simulink model "model_compatible"  (Simulink 7.5)
(part 2 of 2)

  G_23802422_Kernkraftwerk_Isar/RConn2 -- _CN_77697810_380000_CN23802422/RConn2
  G_23802422_Kernkraftwerk_Isar/RConn3 -- _CN_77697810_380000_CN23802422/RConn3
  T_24976300_380000;220000;110000_Umspannwerk_Pleinting/LConn1 -- _CN_77697810_380000_CN_24976300_380000/RConn1
  T_24976300_380000;220000;110000_Umspannwerk_Pleinting/LConn2 -- _CN_77697810_380000_CN_24976300_380000/RConn2
  T_24976300_380000;220000;110000_Umspannwerk_Pleinting/LConn3 -- _CN_77697810_380000_CN_24976300_380000/RConn3
  Nfi_Oh_CN_24158385_220000_CN_26245195_220000/LConn1 -- T_24158385_220000;110000_Umspannwerk_Neufinsing/LConn1 -- Oberbachern___Neufinsing_CN_24158385_220000_CN_18629425_220000/LConn1 -- _CN_24158385_220000_CN_75865676_220000/LConn1 -- Neufinsing___Zolling_CN_24158385_220000_CN29122363/LConn1 -- Neufinsing___Zolling_CN_24158385_220000_CN_133342285_220000/RConn1
  Nfi_Oh_CN_24158385_220000_CN_26245195_220000/LConn2 -- T_24158385_220000;110000_Umspannwerk_Neufinsing/LConn2 -- Oberbachern___Neufinsing_CN_24158385_220000_CN_18629425_220000/LConn2 -- _CN_24158385_220000_CN_75865676_220000/LConn2 -- Neufinsing___Zolling_CN_24158385_220000_CN29122363/LConn2 -- Neufinsing___Zolling_CN_24158385_220000_CN_133342285_220000/RConn2
  Nfi_Oh_CN_24158385_220000_CN_26245195_220000/LConn3 -- T_24158385_220000;110000_Umspannwerk_Neufinsing/LConn3 -- Oberbachern___Neufinsing_CN_24158385_220000_CN_18629425_220000/LConn3 -- _CN_24158385_220000_CN_75865676_220000/LConn3 -- Neufinsing___Zolling_CN_24158385_220000_CN29122363/LConn3 -- Neufinsing___Zolling_CN_24158385_220000_CN_133342285_220000/RConn3
  Nfi_Oh_CN_24158385_220000_CN_26245195_220000/RConn1 -- T_26245195_380000;220000_Umspannwerk_Ottenhofen/RConn1 -- L_26245195/LConn1
  Nfi_Oh_CN_24158385_220000_CN_26245195_220000/RConn2 -- T_26245195_380000;220000_Umspannwerk_Ottenhofen/RConn2 -- L_26245195/LConn2
  Nfi_Oh_CN_24158385_220000_CN_26245195_220000/RConn3 -- T_26245195_380000;220000_Umspannwerk_Ottenhofen/RConn3 -- L_26245195/LConn3
  Oberbachern___Neufinsing_CN_24158385_220000_CN_18629425_220000/RConn1 -- T_18629425_380000;220000;110000_Umspannwerk_Oberbachern/RConn1 -- Oberbrunn___Oberbachern_CN_18629425_220000_CN_24237879_220000/LConn1
  Oberbachern___Neufinsing_CN_24158385_220000_CN_18629425_220000/RConn2 -- T_18629425_380000;220000;110000_Umspannwerk_Oberbachern/RConn2 -- Oberbrunn___Oberbachern_CN_18629425_220000_CN_24237879_220000/LConn2
  Oberbachern___Neufinsing_CN_24158385_220000_CN_18629425_220000/RConn3 -- T_18629425_380000;220000;110000_Umspannwerk_Oberbachern/RConn3 -- Oberbrunn___Oberbachern_CN_18629425_220000_CN_24237879_220000/LConn3
  T_75865676_220000_Umspannwerk_Marienberg/LConn1 -- _CN_24158385_220000_CN_75865676_220000/RConn1
  T_75865676_220000_Umspannwerk_Marienberg/LConn2 -- _CN_24158385_220000_CN_75865676_220000/RConn2
  T_75865676_220000_Umspannwerk_Marienberg/LConn3 -- _CN_24158385_220000_CN_75865676_220000/RConn3
  Neufinsing___Zolling_CN_24158385_220000_CN29122363/RConn1 -- G_29122363_Kraftwerk_Irsching/RConn1 -- _CN_18629425_380000_CN29122363/LConn1 -- Irsching___Raitersaich_CN_24768051_380000_CN29122363/LConn1 -- _CN_137602559_220000_CN29122363/LConn1
  Neufinsing___Zolling_CN_24158385_220000_CN29122363/RConn2 -- G_29122363_Kraftwerk_Irsching/RConn2 -- _CN_18629425_380000_CN29122363/LConn2 -- Irsching___Raitersaich_CN_24768051_380000_CN29122363/LConn2 -- _CN_137602559_220000_CN29122363/LConn2
  Neufinsing___Zolling_CN_24158385_220000_CN29122363/RConn3 -- G_29122363_Kraftwerk_Irsching/RConn3 -- _CN_18629425_380000_CN29122363/LConn3 -- Irsching___Raitersaich_CN_24768051_380000_CN29122363/LConn3 -- _CN_137602559_220000_CN29122363/LConn3
  T_78441561_380000;110000_Umspannwerk_Plattling/LConn1 -- Pleinting___Plattling___Schwandorf_CN_78441561_380000_CN_28956649_380000/LConn1
  T_78441561_380000;110000_Umspannwerk_Plattling/LConn2 -- Pleinting___Plattling___Schwandorf_CN_78441561_380000_CN_28956649_380000/LConn2
  T_78441561_380000;110000_Umspannwerk_Plattling/LConn3 -- Pleinting___Plattling___Schwandorf_CN_78441561_380000_CN_28956649_380000/LConn3
  Pleinting___Plattling___Schwandorf_CN_78441561_380000_CN_28956649_380000/RConn1 -- T_28956649_380000;220000;110000_Schwandorf/LConn1 -- Schwandorf___Etzenricht_CN_29084374_380000_CN_28956649_380000/LConn1
  Pleinting___Plattling___Schwandorf_CN_78441561_380000_CN_28956649_380000/RConn2 -- T_28956649_380000;220000;110000_Schwandorf/LConn2 -- Schwandorf___Etzenricht_CN_29084374_380000_CN_28956649_380000/LConn2
  Pleinting___Plattling___Schwandorf_CN_78441561_380000_CN_28956649_380000/RConn3 -- T_28956649_380000;220000;110000_Schwandorf/LConn3 -- Schwandorf___Etzenricht_CN_29084374_380000_CN_28956649_380000/LConn3
  LU_SIT_CN_24759324_220000_CN_133349218_220000/RConn1 -- T_24759324_220000;110000_Umspannwerk_Sittling/LConn1 -- Altheim___Sittling_CN_24759324_220000_CN_77694901_220000/RConn1 -- IN_SIT_CN_24759324_220000_CN_24768051_220000/LConn1
  LU_SIT_CN_24759324_220000_CN_133349218_220000/RConn2 -- T_24759324_220000;110000_Umspannwerk_Sittling/LConn2 -- Altheim___Sittling_CN_24759324_220000_CN_77694901_220000/RConn2 -- IN_SIT_CN_24759324_220000_CN_24768051_220000/LConn2
  LU_SIT_CN_24759324_220000_CN_133349218_220000/RConn3 -- T_24759324_220000;110000_Umspannwerk_Sittling/LConn3 -- Altheim___Sittling_CN_24759324_220000_CN_77694901_220000/RConn3 -- IN_SIT_CN_24759324_220000_CN_24768051_220000/LConn3
  IN_SIT_CN_24759324_220000_CN_24768051_220000/RConn1 -- T_24768051_380000;220000;110000_Ingolstadt/RConn1 -- Irsching___Raitersaich;Ingolstadt___Raitersaich_CN_24768051_220000_CN_24705761_220000/RConn1
  IN_SIT_CN_24759324_220000_CN_24768051_220000/RConn2 -- T_24768051_380000;220000;110000_Ingolstadt/RConn2 -- Irsching___Raitersaich;Ingolstadt___Raitersaich_CN_24768051_220000_CN_24705761_220000/RConn2
  IN_SIT_CN_24759324_220000_CN_24768051_220000/RConn3 -- T_24768051_380000;220000;110000_Ingolstadt/RConn3 -- Irsching___Raitersaich;Ingolstadt___Raitersaich_CN_24768051_220000_CN_24705761_220000/RConn3
  T_57727006_380000;220000_Schaltanlage_Leupolz/LConn1 -- Leupolz___Oberottmarshausen_CN_57727006_380000_CN_77038371_380000/RConn1
  T_57727006_380000;220000_Schaltanlage_Leupolz/LConn2 -- Leupolz___Oberottmarshausen_CN_57727006_380000_CN_77038371_380000/RConn2
  T_57727006_380000;220000_Schaltanlage_Leupolz/LConn3 -- Leupolz___Oberottmarshausen_CN_57727006_380000_CN_77038371_380000/RConn3
  T_31019937_380000;220000;110000_Vöhringen_LEW/LConn1 -- _CN_31019937_380000_CN_85523877_380000/LConn1
  T_31019937_380000;220000;110000_Vöhringen_LEW/LConn2 -- _CN_31019937_380000_CN_85523877_380000/LConn2
  T_31019937_380000;220000;110000_Vöhringen_LEW/LConn3 -- _CN_31019937_380000_CN_85523877_380000/LConn3
  _CN_31019937_380000_CN_85523877_380000/RConn1 -- T_85523877_380000_Vöhringen_Amprion/LConn1 -- Günzburg_Nord_CN_85523877_380000_CN_24652261_380000/RConn1 -- Günzburg_Nord_CN_85523877_380000_CN_88945213_380000/LConn1
  _CN_31019937_380000_CN_85523877_380000/RConn2 -- T_85523877_380000_Vöhringen_Amprion/LConn2 -- Günzburg_Nord_CN_85523877_380000_CN_24652261_380000/RConn2 -- Günzburg_Nord_CN_85523877_380000_CN_88945213_380000/LConn2
  _CN_31019937_380000_CN_85523877_380000/RConn3 -- T_85523877_380000_Vöhringen_Amprion/LConn3 -- Günzburg_Nord_CN_85523877_380000_CN_24652261_380000/RConn3 -- Günzburg_Nord_CN_85523877_380000_CN_88945213_380000/LConn3
  T_31019939_380000;110000_Gundremmingen/LConn1 -- _CN_31019939_380000_CN_88945213_380000/LConn1
  T_31019939_380000;110000_Gundremmingen/LConn2 -- _CN_31019939_380000_CN_88945213_380000/LConn2
  T_31019939_380000;110000_Gundremmingen/LConn3 -- _CN_31019939_380000_CN_88945213_380000/LConn3
  _CN_31019939_380000_CN_88945213_380000/RConn1 -- T_88945213_380000_Umspannwerk_Gundelfingen/LConn1 -- _CN_88945213_380000_CN31023006/LConn1 -- Günzburg_Nord_CN_85523877_380000_CN_88945213_380000/RConn1
  _CN_31019939_380000_CN_88945213_380000/RConn2 -- T_88945213_380000_Umspannwerk_Gundelfingen/LConn2 -- _CN_88945213_380000_CN31023006/LConn2 -- Günzburg_Nord_CN_85523877_380000_CN_88945213_380000/RConn2
  _CN_31019939_380000_CN_88945213_380000/RConn3 -- T_88945213_380000_Umspannwerk_Gundelfingen/LConn3 -- _CN_88945213_380000_CN31023006/LConn3 -- Günzburg_Nord_CN_85523877_380000_CN_88945213_380000/RConn3
  OBA___MZ_CN_18629425_380000_CN_23907283_380000/LConn1 -- T_18629425_380000;220000;110000_Umspannwerk_Oberbachern/LConn1 -- _CN_18629425_380000_CN_26245195_380000/RConn1 -- _CN_18629425_380000_CN29122363/RConn1 -- Meitingen___Oberbachern_CN_18629425_380000_CN_24652261_380000/RConn1
  OBA___MZ_CN_18629425_380000_CN_23907283_380000/LConn2 -- T_18629425_380000;220000;110000_Umspannwerk_Oberbachern/LConn2 -- _CN_18629425_380000_CN_26245195_380000/RConn2 -- _CN_18629425_380000_CN29122363/RConn2 -- Meitingen___Oberbachern_CN_18629425_380000_CN_24652261_380000/RConn2
  OBA___MZ_CN_18629425_380000_CN_23907283_380000/LConn3 -- T_18629425_380000;220000;110000_Umspannwerk_Oberbachern/LConn3 -- _CN_18629425_380000_CN_26245195_380000/RConn3 -- _CN_18629425_380000_CN29122363/RConn3 -- Meitingen___Oberbachern_CN_18629425_380000_CN_24652261_380000/RConn3
  T_23907283_380000;110000_Hauptumspannwerk_Menzing/LConn1 -- OBA___MZ_CN_18629425_380000_CN_23907283_380000/RConn1
  T_23907283_380000;110000_Hauptumspannwerk_Menzing/LConn2 -- OBA___MZ_CN_18629425_380000_CN_23907283_380000/RConn2
  T_23907283_380000;110000_Hauptumspannwerk_Menzing/LConn3 -- OBA___MZ_CN_18629425_380000_CN_23907283_380000/RConn3
  Oberbrunn___Oberbachern_CN_18629425_220000_CN_24237879_220000/RConn1 -- T_24237879_220000;110000_Umspannwerk_Oberbrunn/LConn1 -- OBR_KR_SSI_CN_24237879_220000_CN252655527/LConn1
  Oberbrunn___Oberbachern_CN_18629425_220000_CN_24237879_220000/RConn2 -- T_24237879_220000;110000_Umspannwerk_Oberbrunn/LConn2 -- OBR_KR_SSI_CN_24237879_220000_CN252655527/LConn2
  Oberbrunn___Oberbachern_CN_18629425_220000_CN_24237879_220000/RConn3 -- T_24237879_220000;110000_Umspannwerk_Oberbrunn/LConn3 -- OBR_KR_SSI_CN_24237879_220000_CN252655527/LConn3
  T_90807341_220000;110000_Umspannwerk_Kempten_Au/LConn1 -- _CN_90807341_220000_CN_46766896_220000/RConn1
  T_90807341_220000;110000_Umspannwerk_Kempten_Au/LConn2 -- _CN_90807341_220000_CN_46766896_220000/RConn2
  T_90807341_220000;110000_Umspannwerk_Kempten_Au/LConn3 -- _CN_90807341_220000_CN_46766896_220000/RConn3
  T_5404079_380000;110000_Föhring/LConn1 -- OH_FO_CN_5404079_380000_CN_26245195_380000/RConn1
  T_5404079_380000;110000_Föhring/LConn2 -- OH_FO_CN_5404079_380000_CN_26245195_380000/RConn2
  T_5404079_380000;110000_Föhring/LConn3 -- OH_FO_CN_5404079_380000_CN_26245195_380000/RConn3
  OBR_KR_SSI_CN_24237879_220000_CN252655527/RConn1 -- G_252655527_Stauwehr_Krün/RConn1 -- _CN_68532663_220000_CN252655527/LConn1
  OBR_KR_SSI_CN_24237879_220000_CN252655527/RConn2 -- G_252655527_Stauwehr_Krün/RConn2 -- _CN_68532663_220000_CN252655527/LConn2
  OBR_KR_SSI_CN_24237879_220000_CN252655527/RConn3 -- G_252655527_Stauwehr_Krün/RConn3 -- _CN_68532663_220000_CN252655527/LConn3
  Irsching___Raitersaich;Ingolstadt___Raitersaich_CN_24768051_380000_CN_24705761_380000/RConn1 -- T_24768051_380000;220000;110000_Ingolstadt/LConn1 -- Irsching___Raitersaich_CN_24768051_380000_CN29122363/RConn1
  Irsching___Raitersaich;Ingolstadt___Raitersaich_CN_24768051_380000_CN_24705761_380000/RConn2 -- T_24768051_380000;220000;110000_Ingolstadt/LConn2 -- Irsching___Raitersaich_CN_24768051_380000_CN29122363/RConn2
  Irsching___Raitersaich;Ingolstadt___Raitersaich_CN_24768051_380000_CN_24705761_380000/RConn3 -- T_24768051_380000;220000;110000_Ingolstadt/LConn3 -- Irsching___Raitersaich_CN_24768051_380000_CN29122363/RConn3
  G_31023006_/RConn1 -- _CN_88945213_380000_CN31023006/RConn1
  G_31023006_/RConn2 -- _CN_88945213_380000_CN31023006/RConn2
  G_31023006_/RConn3 -- _CN_88945213_380000_CN31023006/RConn3
  T_68532663_220000;110000_Umspannwerk_Krün/LConn1 -- _CN_68532663_220000_CN252655527/RConn1
  T_68532663_220000;110000_Umspannwerk_Krün/LConn2 -- _CN_68532663_220000_CN252655527/RConn2
  T_68532663_220000;110000_Umspannwerk_Krün/LConn3 -- _CN_68532663_220000_CN252655527/RConn3
  T_276236628_220000;110000_Schweinfurt/LConn1 -- _CN_276236628_220000_CN_24715381_220000/LConn1
  T_276236628_220000;110000_Schweinfurt/LConn2 -- _CN_276236628_220000_CN_24715381_220000/LConn2
  T_276236628_220000;110000_Schweinfurt/LConn3 -- _CN_276236628_220000_CN_24715381_220000/LConn3
  _CN_276236628_220000_CN_24715381_220000/RConn1 -- T_24715381_380000;220000;110000_Umspannwerk_Bergrheinfeld/RConn1 -- _CN_24705761_220000_CN_24715381_220000/RConn1
  _CN_276236628_220000_CN_24715381_220000/RConn2 -- T_24715381_380000;220000;110000_Umspannwerk_Bergrheinfeld/RConn2 -- _CN_24705761_220000_CN_24715381_220000/RConn2
  _CN_276236628_220000_CN_24715381_220000/RConn3 -- T_24715381_380000;220000;110000_Umspannwerk_Bergrheinfeld/RConn3 -- _CN_24705761_220000_CN_24715381_220000/RConn3
  Etzenricht___Mechlenreuth___Redwitz_CN_29084374_380000_CN_93341407_380000/RConn1 -- T_29084374_380000;110000_Umspannwerk_Etzenricht/LConn1 -- Schwandorf___Etzenricht_CN_29084374_380000_CN_28956649_380000/RConn1
  Etzenricht___Mechlenreuth___Redwitz_CN_29084374_380000_CN_93341407_380000/RConn2 -- T_29084374_380000;110000_Umspannwerk_Etzenricht/LConn2 -- Schwandorf___Etzenricht_CN_29084374_380000_CN_28956649_380000/RConn2
  Etzenricht___Mechlenreuth___Redwitz_CN_29084374_380000_CN_93341407_380000/RConn3 -- T_29084374_380000;110000_Umspannwerk_Etzenricht/LConn3 -- Schwandorf___Etzenricht_CN_29084374_380000_CN_28956649_380000/RConn3
  T_93341407_380000;220000;110000_Umspannwerk_Mechlenreuth/RConn1 -- MH___SD_CN_93341407_220000_CN_28956649_220000/RConn1
  T_93341407_380000;220000;110000_Umspannwerk_Mechlenreuth/RConn2 -- MH___SD_CN_93341407_220000_CN_28956649_220000/RConn2
  T_93341407_380000;220000;110000_Umspannwerk_Mechlenreuth/RConn3 -- MH___SD_CN_93341407_220000_CN_28956649_220000/RConn3
  T_91080806_220000;110000_Umspannwerk_Pirach/LConn1 -- _CN_91080806_220000_CN167578660/RConn1
  T_91080806_220000;110000_Umspannwerk_Pirach/LConn2 -- _CN_91080806_220000_CN167578660/RConn2
  T_91080806_220000;110000_Umspannwerk_Pirach/LConn3 -- _CN_91080806_220000_CN167578660/RConn3
  T_137602559_380000;220000;110000_Irsching/LConn1 -- _CN_137602559_220000_CN29122363/RConn1
  T_137602559_380000;220000;110000_Irsching/LConn2 -- _CN_137602559_220000_CN29122363/RConn2
  T_137602559_380000;220000;110000_Irsching/LConn3 -- _CN_137602559_220000_CN29122363/RConn3
  T_108797675_380000_Grafenrheinfeld/RConn1 -- L_108797675/LConn1
  T_108797675_380000_Grafenrheinfeld/RConn2 -- L_108797675/LConn2
  T_108797675_380000_Grafenrheinfeld/RConn3 -- L_108797675/LConn3
  T_24715381_380000;220000;110000_Umspannwerk_Bergrheinfeld/RConn4 -- L_24715381/LConn1
  T_24715381_380000;220000;110000_Umspannwerk_Bergrheinfeld/RConn5 -- L_24715381/LConn2
  T_24715381_380000;220000;110000_Umspannwerk_Bergrheinfeld/RConn6 -- L_24715381/LConn3
  T_24758329_380000;110000_Umspannwerk_Eltmann/RConn1 -- L_24758329/LConn1
  T_24758329_380000;110000_Umspannwerk_Eltmann/RConn2 -- L_24758329/LConn2
  T_24758329_380000;110000_Umspannwerk_Eltmann/RConn3 -- L_24758329/LConn3
  T_24757833_380000_Umspannwerk_Oberhaid/RConn1 -- L_24757833/LConn1
  T_24757833_380000_Umspannwerk_Oberhaid/RConn2 -- L_24757833/LConn2
  T_24757833_380000_Umspannwerk_Oberhaid/RConn3 -- L_24757833/LConn3
  T_24757393__Umspannwerk_Würgau/RConn1 -- L_24757393/LConn1
  T_24757393__Umspannwerk_Würgau/RConn2 -- L_24757393/LConn2
  T_24757393__Umspannwerk_Würgau/RConn3 -- L_24757393/LConn3
  T_24705761_380000;220000;110000_Umspannwerk_Raitersaich/RConn4 -- L_24705761/LConn1
  T_24705761_380000;220000;110000_Umspannwerk_Raitersaich/RConn5 -- L_24705761/LConn2
  T_24705761_380000;220000;110000_Umspannwerk_Raitersaich/RConn6 -- L_24705761/LConn3
  T_28613721_380000;110000_Kriegenbrunn/RConn1 -- L_28613721/LConn1
  T_28613721_380000;110000_Kriegenbrunn/RConn2 -- L_28613721/LConn2
  T_28613721_380000;110000_Kriegenbrunn/RConn3 -- L_28613721/LConn3
  T_24757392_380000;110000_Umspannwerk_Redwitz/RConn1 -- L_24757392/LConn1
  T_24757392_380000;110000_Umspannwerk_Redwitz/RConn2 -- L_24757392/LConn2
  T_24757392_380000;110000_Umspannwerk_Redwitz/RConn3 -- L_24757392/LConn3
  T_55069713_380000;220000;110000_Umspannwerk_Aschaffenburg/RConn4 -- L_55069713/LConn1
  T_55069713_380000;220000;110000_Umspannwerk_Aschaffenburg/RConn5 -- L_55069713/LConn2
  T_55069713_380000;220000;110000_Umspannwerk_Aschaffenburg/RConn6 -- L_55069713/LConn3
  T_232833796_220000_/RConn1 -- L_232833796/LConn1
  T_232833796_220000_/RConn2 -- L_232833796/LConn2
  T_232833796_220000_/RConn3 -- L_232833796/LConn3
  T_133342285_220000;110000_Zolling___Irsching/RConn1 -- L_133342285/LConn1
  T_133342285_220000;110000_Zolling___Irsching/RConn2 -- L_133342285/LConn2
  T_133342285_220000;110000_Zolling___Irsching/RConn3 -- L_133342285/LConn3
  T_30613895_380000;220000;110000_Umspannwerk_Oberottmarshausen/RConn4 -- L_30613895/LConn1
  T_30613895_380000;220000;110000_Umspannwerk_Oberottmarshausen/RConn5 -- L_30613895/LConn2
  T_30613895_380000;220000;110000_Umspannwerk_Oberottmarshausen/RConn6 -- L_30613895/LConn3
  T_77038371_380000;110000_Umspannwerk_Bidingen_Nr__697_S/RConn1 -- L_77038371/LConn1
  T_77038371_380000;110000_Umspannwerk_Bidingen_Nr__697_S/RConn2 -- L_77038371/LConn2
  T_77038371_380000;110000_Umspannwerk_Bidingen_Nr__697_S/RConn3 -- L_77038371/LConn3
  T_31019937_380000;220000;110000_Vöhringen_LEW/RConn4 -- L_31019937/LConn1
  T_31019937_380000;220000;110000_Vöhringen_LEW/RConn5 -- L_31019937/LConn2
  T_31019937_380000;220000;110000_Vöhringen_LEW/RConn6 -- L_31019937/LConn3
  T_24652261_380000_Station_Meitingen/RConn1 -- L_24652261/LConn1
  T_24652261_380000_Station_Meitingen/RConn2 -- L_24652261/LConn2
  T_24652261_380000_Station_Meitingen/RConn3 -- L_24652261/LConn3
  T_53378027_380000;110000_Umspannwerk_Lechhausen;_Übernahmestation_Lechhausen/RConn1 -- L_53378027/LConn1
  T_53378027_380000;110000_Umspannwerk_Lechhausen;_Übernahmestation_Lechhausen/RConn2 -- L_53378027/LConn2
  T_53378027_380000;110000_Umspannwerk_Lechhausen;_Übernahmestation_Lechhausen/RConn3 -- L_53378027/LConn3
  T_27200252_220000;110000_Umspannstation_Irsingen/RConn1 -- L_27200252/LConn1
  T_27200252_220000;110000_Umspannstation_Irsingen/RConn2 -- L_27200252/LConn2
  T_27200252_220000;110000_Umspannstation_Irsingen/RConn3 -- L_27200252/LConn3
  T_25487161_220000;110000_Umspannwerk_Memmingen/RConn1 -- L_25487161/LConn1
  T_25487161_220000;110000_Umspannwerk_Memmingen/RConn2 -- L_25487161/LConn2
  T_25487161_220000;110000_Umspannwerk_Memmingen/RConn3 -- L_25487161/LConn3
  T_46766896_220000_Schaltwerk_Kempten/RConn1 -- L_46766896/LConn1
  T_46766896_220000_Schaltwerk_Kempten/RConn2 -- L_46766896/LConn2
  T_46766896_220000_Schaltwerk_Kempten/RConn3 -- L_46766896/LConn3
  T_34414970_220000;110000_Umspannwerk_Rauhenzell/RConn1 -- L_34414970/LConn1
  T_34414970_220000;110000_Umspannwerk_Rauhenzell/RConn2 -- L_34414970/LConn2
  T_34414970_220000;110000_Umspannwerk_Rauhenzell/RConn3 -- L_34414970/LConn3
  T_91086220_220000_Umspannwerk_Simbach/RConn1 -- L_91086220/LConn1
  T_91086220_220000_Umspannwerk_Simbach/RConn2 -- L_91086220/LConn2
  T_91086220_220000_Umspannwerk_Simbach/RConn3 -- L_91086220/LConn3
  T_24976300_380000;220000;110000_Umspannwerk_Pleinting/RConn4 -- L_24976300/LConn1
  T_24976300_380000;220000;110000_Umspannwerk_Pleinting/RConn5 -- L_24976300/LConn2
  T_24976300_380000;220000;110000_Umspannwerk_Pleinting/RConn6 -- L_24976300/LConn3
  T_77694901_220000;110000_Umspannwerk_Altheim/RConn1 -- L_77694901/LConn1
  T_77694901_220000;110000_Umspannwerk_Altheim/RConn2 -- L_77694901/LConn2
  T_77694901_220000;110000_Umspannwerk_Altheim/RConn3 -- L_77694901/LConn3
  T_29417741_220000_Umspannwerk_Regensburg/RConn1 -- L_29417741/LConn1
  T_29417741_220000_Umspannwerk_Regensburg/RConn2 -- L_29417741/LConn2
  T_29417741_220000_Umspannwerk_Regensburg/RConn3 -- L_29417741/LConn3
  T_28956649_380000;220000;110000_Schwandorf/RConn4 -- L_28956649/LConn1
  T_28956649_380000;220000;110000_Schwandorf/RConn5 -- L_28956649/LConn2
  T_28956649_380000;220000;110000_Schwandorf/RConn6 -- L_28956649/LConn3
  T_76246159_380000;110000_Umspannwerk_Meitingen/RConn1 -- L_76246159/LConn1
  T_76246159_380000;110000_Umspannwerk_Meitingen/RConn2 -- L_76246159/LConn2
  T_76246159_380000;110000_Umspannwerk_Meitingen/RConn3 -- L_76246159/LConn3
  T_93341407_380000;220000;110000_Umspannwerk_Mechlenreuth/RConn4 -- L_93341407/LConn1
  T_93341407_380000;220000;110000_Umspannwerk_Mechlenreuth/RConn5 -- L_93341407/LConn2
  T_93341407_380000;220000;110000_Umspannwerk_Mechlenreuth/RConn6 -- L_93341407/LConn3
  T_24765111_220000;110000_Umspannwerk_Trennfeld/RConn1 -- L_24765111/LConn1
  T_24765111_220000;110000_Umspannwerk_Trennfeld/RConn2 -- L_24765111/LConn2
  T_24765111_220000;110000_Umspannwerk_Trennfeld/RConn3 -- L_24765111/LConn3
  T_133349218_220000;110000_Umspannwerk_Ludersheim/RConn1 -- L_133349218/LConn1
  T_133349218_220000;110000_Umspannwerk_Ludersheim/RConn2 -- L_133349218/LConn2
  T_133349218_220000;110000_Umspannwerk_Ludersheim/RConn3 -- L_133349218/LConn3
  T_77697810_380000_Isar/RConn1 -- L_77697810/LConn1
  T_77697810_380000_Isar/RConn2 -- L_77697810/LConn2
  T_77697810_380000_Isar/RConn3 -- L_77697810/LConn3
  T_24158385_220000;110000_Umspannwerk_Neufinsing/RConn1 -- L_24158385/LConn1
  T_24158385_220000;110000_Umspannwerk_Neufinsing/RConn2 -- L_24158385/LConn2
  T_24158385_220000;110000_Umspannwerk_Neufinsing/RConn3 -- L_24158385/LConn3
  T_18629425_380000;220000;110000_Umspannwerk_Oberbachern/RConn4 -- L_18629425/LConn1
  T_18629425_380000;220000;110000_Umspannwerk_Oberbachern/RConn5 -- L_18629425/LConn2
  T_18629425_380000;220000;110000_Umspannwerk_Oberbachern/RConn6 -- L_18629425/LConn3
  T_75865676_220000_Umspannwerk_Marienberg/RConn1 -- L_75865676/LConn1
  T_75865676_220000_Umspannwerk_Marienberg/RConn2 -- L_75865676/LConn2
  T_75865676_220000_Umspannwerk_Marienberg/RConn3 -- L_75865676/LConn3
  T_78441561_380000;110000_Umspannwerk_Plattling/RConn1 -- L_78441561/LConn1
  T_78441561_380000;110000_Umspannwerk_Plattling/RConn2 -- L_78441561/LConn2
  T_78441561_380000;110000_Umspannwerk_Plattling/RConn3 -- L_78441561/LConn3
  T_24759324_220000;110000_Umspannwerk_Sittling/RConn1 -- L_24759324/LConn1
  T_24759324_220000;110000_Umspannwerk_Sittling/RConn2 -- L_24759324/LConn2
  T_24759324_220000;110000_Umspannwerk_Sittling/RConn3 -- L_24759324/LConn3
  T_24768051_380000;220000;110000_Ingolstadt/RConn4 -- L_24768051/LConn1
  T_24768051_380000;220000;110000_Ingolstadt/RConn5 -- L_24768051/LConn2
  T_24768051_380000;220000;110000_Ingolstadt/RConn6 -- L_24768051/LConn3
  T_85523877_380000_Vöhringen_Amprion/RConn1 -- L_85523877/LConn1
  T_85523877_380000_Vöhringen_Amprion/RConn2 -- L_85523877/LConn2
  T_85523877_380000_Vöhringen_Amprion/RConn3 -- L_85523877/LConn3
  T_31019939_380000;110000_Gundremmingen/RConn1 -- L_31019939/LConn1
  T_31019939_380000;110000_Gundremmingen/RConn2 -- L_31019939/LConn2
  T_31019939_380000;110000_Gundremmingen/RConn3 -- L_31019939/LConn3
  T_88945213_380000_Umspannwerk_Gundelfingen/RConn1 -- L_88945213/LConn1
  T_88945213_380000_Umspannwerk_Gundelfingen/RConn2 -- L_88945213/LConn2
  T_88945213_380000_Umspannwerk_Gundelfingen/RConn3 -- L_88945213/LConn3
  T_23907283_380000;110000_Hauptumspannwerk_Menzing/RConn1 -- L_23907283/LConn1
  T_23907283_380000;110000_Hauptumspannwerk_Menzing/RConn2 -- L_23907283/LConn2
  T_23907283_380000;110000_Hauptumspannwerk_Menzing/RConn3 -- L_23907283/LConn3
  T_24237879_220000;110000_Umspannwerk_Oberbrunn/RConn1 -- L_24237879/LConn1
  T_24237879_220000;110000_Umspannwerk_Oberbrunn/RConn2 -- L_24237879/LConn2
  T_24237879_220000;110000_Umspannwerk_Oberbrunn/RConn3 -- L_24237879/LConn3
  T_90807341_220000;110000_Umspannwerk_Kempten_Au/RConn1 -- L_90807341/LConn1
  T_90807341_220000;110000_Umspannwerk_Kempten_Au/RConn2 -- L_90807341/LConn2
  T_90807341_220000;110000_Umspannwerk_Kempten_Au/RConn3 -- L_90807341/LConn3
  T_5404079_380000;110000_Föhring/RConn1 -- L_5404079/LConn1
  T_5404079_380000;110000_Föhring/RConn2 -- L_5404079/LConn2
  T_5404079_380000;110000_Föhring/RConn3 -- L_5404079/LConn3
  T_68532663_220000;110000_Umspannwerk_Krün/RConn1 -- L_68532663/LConn1
  T_68532663_220000;110000_Umspannwerk_Krün/RConn2 -- L_68532663/LConn2
  T_68532663_220000;110000_Umspannwerk_Krün/RConn3 -- L_68532663/LConn3
  T_276236628_220000;110000_Schweinfurt/RConn1 -- L_276236628/LConn1
  T_276236628_220000;110000_Schweinfurt/RConn2 -- L_276236628/LConn2
  T_276236628_220000;110000_Schweinfurt/RConn3 -- L_276236628/LConn3
  T_29084374_380000;110000_Umspannwerk_Etzenricht/RConn1 -- L_29084374/LConn1
  T_29084374_380000;110000_Umspannwerk_Etzenricht/RConn2 -- L_29084374/LConn2
  T_29084374_380000;110000_Umspannwerk_Etzenricht/RConn3 -- L_29084374/LConn3
  T_91080806_220000;110000_Umspannwerk_Pirach/RConn1 -- L_91080806/LConn1
  T_91080806_220000;110000_Umspannwerk_Pirach/RConn2 -- L_91080806/LConn2
  T_91080806_220000;110000_Umspannwerk_Pirach/RConn3 -- L_91080806/LConn3
  T_137602559_380000;220000;110000_Irsching/RConn1 -- L_137602559/LConn1
  T_137602559_380000;220000;110000_Irsching/RConn2 -- L_137602559/LConn2
  T_137602559_380000;220000;110000_Irsching/RConn3 -- L_137602559/LConn3
